simulink model "hinfcontroller"  (R2017b)
settings: Solver=VariableStepAuto  StartTime=0.0  StopTime=10  RelTol=1e-3
values from neighbouring files (symbols this model uses):
  x0 = [0.51*pi,0,0.5*pi,0]    [Nonlinearequations.m]    (also in controllerData3.m = [-0.6*pi 0 -0.4*pi 0]; linearizeM.m = [-0.51*pi,0,-0.5*pi,0])
undefined symbols (not defined in the file or in its folder): Ak, Bk, Ck, Dk
settings Model: Creator=geert  LastModifiedBy=geert

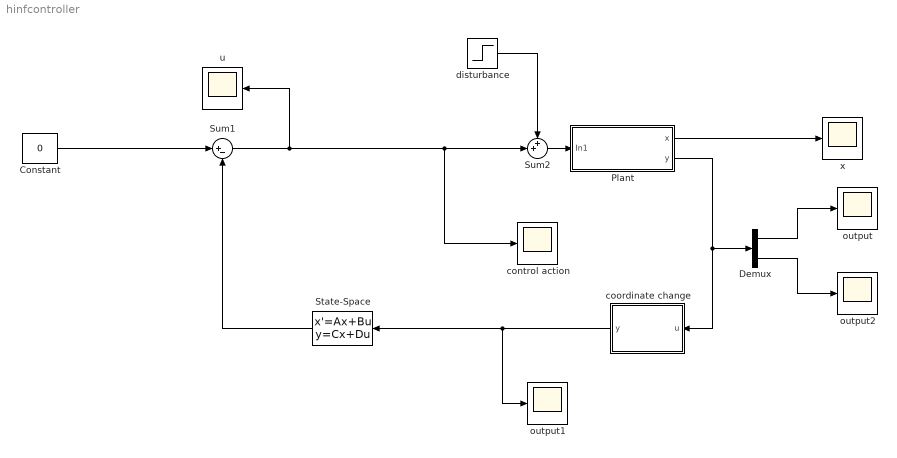
== system hinfcontroller ==
  Constant : Constant  Value=0
  Demux : Demux  Outputs=2
  Plant : Subsystem
  State-Space : StateSpace  A=Ak  B=Bk  C=Ck  D=Dk  InitialCondition=0
  Sum1 : Sum  Inputs=|+-
  Sum2 : Sum  Inputs=++|
  control action : Scope
  coordinate change : MATLAB Function  TreatAsAtomicUnit=on
  disturbance : Step  Time=5  After=0  SampleTime=0
  output : Scope
  output1 : Scope
  output2 : Scope
  u : Scope
  x : Scope
  wires:
  Sum1/1 -> control action/1, Sum2/2, u/1
  Plant/1(x) -> x/1
  Constant/1 -> Sum1/1
  Plant/2(y) -> Demux/1, coordinate change/1(u)
  disturbance/1 -> Sum2/1
  Sum2/1 -> Plant/1(In1)
  coordinate change/1(y) -> output1/1, State-Space/1
  State-Space/1 -> Sum1/2
  Demux/1 -> output/1
  Demux/2 -> output2/1

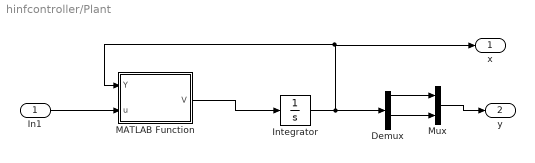
== system hinfcontroller/Plant ==
  In1 : Inport
  Demux : Demux
  Integrator : Integrator  InitialCondition=x0
  MATLAB Function : MATLAB Function  TreatAsAtomicUnit=on
  Mux : Mux  Inputs=2
  x : Outport
  y : Outport  Port=2
  wires:
  Integrator/1 -> Demux/1, x/1, MATLAB Function/1(Y)
  In1/1 -> MATLAB Function/2(u)
  MATLAB Function/1(V) -> Integrator/1
  Demux/1 -> Mux/1
  Demux/3 -> Mux/2
  Mux/1 -> y/1

== matlab function hinfcontroller/coordinate change ==
  data: u input; y output
function y = fcn(u)

y = u + 0.5*pi;

== matlab function hinfcontroller/Plant/MATLAB Function ==
  data: Y input; u input; V output
function V = M(Y,u)
%M
%    V = M(Y,U)

%    This function was generated by the Symbolic Math Toolbox version 8.0.
%    09-May-2018 10:56:52

t3 = Y(1);
t4 = Y(3);
t5 = t3-t4;
t2 = cos(t5);
t6 = t2.^2;
t7 = t6.*7.29e-8;
t8 = t7-8.854411999999999e-6;
t9 = 1.0./t8;
t10 = Y(2);
t11 = Y(4);
t12 = cos(t4);
t13 = cos(t3);
t14 = sin(t5);
t15 = t10.^2;
t16 = t3.*2.0;
t17 = t4.*-2.0+t16;
t18 = sin(t17);
t19 = t11.^2;
V = [t10;t9.*t10.*7.649599999999999e-6+t9.*(t13.*1.013074776e-3-t2.*t12.*4.449816e-5)-t2.*t9.*t11.*9.45e-5+t9.*t14.*t19.*1.032696e-5+t9.*t15.*t18.*3.645000000000001e-8+t2.*t9.*u.*4.86e-4;t11;t9.*(t12.*3.8153052e-5-t2.*t13.*7.15149e-6)+t9.*t11.*8.1025e-5-t9.*u.*4.167e-4-t2.*t9.*t10.*5.4e-8-t9.*t14.*t15.*6.2505e-8-t9.*t18.*t19.*3.645000000000001e-8];
